simulink model "testmodel_5_clean"  (R2018b)
settings: Solver=VariableStepAuto  StartTime=0.0  StopTime=20  RelTol=1e-3
values from neighbouring files (symbols this model uses):
  Brain_gain = 3    [Model_versie_5_clean.m]
  Hoeksnelheid = 60    [Model_versie_1.m]    (also in Model_versie_5_clean.m = 200)
  k_1 = 1/K_g    (= 1.26582278481)    [Model_versie_1.m]    (also in Model_versie_5_clean.m)
  mu = 1.5    [Model_versie_1.m]    (also in Model_versie_5_clean.m = B_g/(2*sqrt(K_g*J_g)))
  Saccade_gain = 6    [Model_versie_5_clean.m]
  Time_delay = 0.00    (= 0)    [Model_versie_1.m]    (also in Model_versie_5_clean.m = 0.01)
  wn = 10    [Model_versie_1.m]    (also in Model_versie_5_clean.m = sqrt(K_g/J_g))
libraries: dspswit3 x1, simulink x1
settings Model: Creator=janwi  LastModifiedBy=janwi
settings SimscapeCC: SimscapeLogType=all

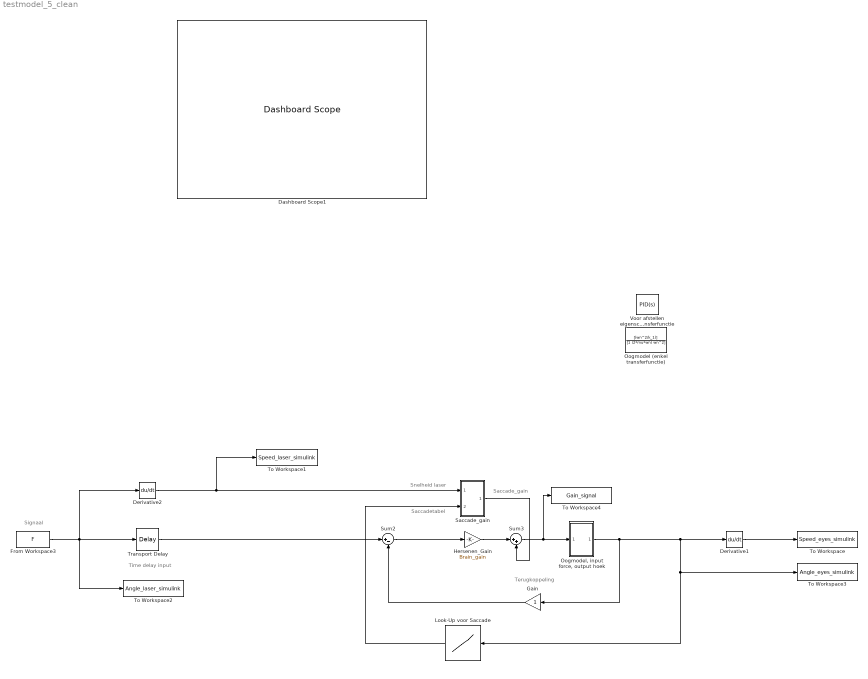
== system testmodel_5_clean ==
  note: Saccade_gain
  note: Saccadetabel
  note: Snelheid laser
  note: Terugkoppeling
  note: Signaal
  note: Time delay input
  Dashboard Scope1 : DashboardScope  WebBlockId=93
  Derivative1 : Derivative  CoefficientInTFapproximation=1
  Derivative2 : Derivative  CoefficientInTFapproximation=1
  From Workspace3 : FromWorkspace  VariableName=F  SampleTime=0
  Gain : Gain
  Hersenen_Gain : Gain  Gain=Brain_gain
  Look-Up voor Saccade : Lookup_n-D  NumberOfTableDimensions=1  BreakpointsForDimension1=[-34 -17 0 17 34]  Table=[1 2 3 2 1]  InternalRulePriority=Speed  RndMeth=Simplest  InputSameDT=on
  Oogmodel (enkel transferfunctie) : TransferFcn  Numerator=[(wn^2/k_1)]  Denominator=[1 (2*mu*wn) wn^2]
  "Oogmodel, input force, output hoek" : Subsystem
  Saccade_gain : Subsystem
  Sum2 : Sum  Inputs=|+-
  Sum3 : Sum  Inputs=|++
  To Workspace : ToWorkspace  VariableName=Speed_eyes_simulink  SampleTime=1e-3
      settings: Save2DSignal=2-D array (concatenate along first dimension)
  To Workspace1 : ToWorkspace  VariableName=Speed_laser_simulink  SampleTime=1e-3
      settings: Save2DSignal=2-D array (concatenate along first dimension)
  To Workspace2 : ToWorkspace  VariableName=Angle_laser_simulink  SampleTime=1e-3
      settings: Save2DSignal=2-D array (concatenate along first dimension)
  To Workspace3 : ToWorkspace  VariableName=Angle_eyes_simulink  SampleTime=1e-3
      settings: Save2DSignal=2-D array (concatenate along first dimension)
  To Workspace4 : ToWorkspace  VariableName=Gain_signal  SampleTime=1e-3
      settings: Save2DSignal=2-D array (concatenate along first dimension)
  Transport Delay : TransportDelay  DelayTime=Time_delay  InitialOutput=1
  Voor afstellen eigenschappen transferfunctie : simulink/Continuous/PID Controller  Controller=PID  Form=Parallel  TimeDomain=Continuous-time  SampleTime=-1  IntegratorMethod=Forward Euler  FilterMethod=Forward Euler  ControllerParametersSource=internal  P=2.20015768194357  I=166.043688229309  D=-0.000180470989757824  UseFilter=on  N=12191.1986236458  TunerSelectOption=Transfer Function Based (PID Tuner App)  InitialConditionSource=internal  InitialConditionForIntegrator=0  InitialConditionForFilter=0  DifferentiatorICPrevScaledInput=0  ExternalReset=none  TrackingMode=off  Kt=1  LimitOutput=off  UpperSaturationLimit=inf  LowerSaturationLimit=-inf  LinearizeAsGain=on  AntiWindupMode=none  Kb=1  POutMin=[]  POutMax=[]  IOutMin=[]  IOutMax=[]  DOutMin=[]  DOutMax=[]  NOutMin=[]  NOutMax=[]  SumOutMin=[]  SumOutMax=[]  SaturationOutMin=[]  SaturationOutMax=[]  PParamMin=[]  PParamMax=[]  IParamMin=[]  IParamMax=[]  DParamMin=[]  DParamMax=[]  NParamMin=[]  NParamMax=[]  KbParamMin=[]  KbParamMax=[]  KtParamMin=[]  KtParamMax=[]  KbOutMin=[]  KbOutMax=[]  KtOutMin=[]  KtOutMax=[]  IntegratorOutMin=[]  IntegratorOutMax=[]  FilterOutMin=[]  FilterOutMax=[]  SumI1OutMin=[]  SumI1OutMax=[]  SumI2OutMin=[]  SumI2OutMax=[]  SumI3OutMin=[]  SumI3OutMax=[]  SumI4OutMin=[]  SumI4OutMax=[]  SumDOutMin=[]  SumDOutMax=[]  DifferentiatorOutMin=[]  DifferentiatorOutMax=[]  FilterDiffOutCoefMin=[]  FilterDiffOutCoefMax=[]  ReciprocalOutMin=[]  ReciprocalOutMax=[]  SumDenOutMin=[]  SumDenOutMax=[]  SumNumOutMin=[]  SumNumOutMax=[]  DivideOutMin=[]  DivideOutMax=[]  IntegratorContinuousStateAttributes=''  IntegratorStateMustResolveToSignalObject=off  IntegratorRTWStateStorageClass=Auto  FilterContinuousStateAttributes=''  FilterStateMustResolveToSignalObject=off  FilterRTWStateStorageClass=Auto  ParallelPVariant=InternalParameters  IdealPVariant=Disabled  IVariant=InternalParameters  DVariant=InternalParameters  IntegratorVariant=Continuous  SatVariant=Disabled  AWVariant=Passthrough  PCopyVariant=Disabled  TRVariant=Disabled  FdbkBlocksVariant=Forward  IdealPFdbkVariant=Disabled  SatFdbkVariant=Disabled  DerivativeFilterVariant=ContFilter  NVariant=InternalParameters  NCopyVariant=Disabled  FilterICVariant=InternalICsFilter  IntegratorICVariant=InternalICs  ExternalResetVariant=Disabled  TRSumVariant=Passthrough  SumFdbkVariant=Disabled  SumVariant=Sum_PID
  wires:
  From Workspace3/1 -> To Workspace2/1, Transport Delay/1, Derivative2/1
  Derivative2/1 -> To Workspace1/1, Saccade_gain/1(In3)
  Transport Delay/1 -> Sum2/1
  Sum2/1 -> Hersenen_Gain/1
  "Oogmodel, input force, output hoek"/1(Out2) -> Look-Up voor Saccade/1, To Workspace3/1, Derivative1/1, Gain/1
  Derivative1/1 -> To Workspace/1
  Gain/1 -> Sum2/2
  Hersenen_Gain/1 -> Sum3/1
  Sum3/1 -> To Workspace4/1, "Oogmodel, input force, output hoek"/1(In1)
  Look-Up voor Saccade/1 -> Saccade_gain/2(In6)
  Saccade_gain/1(Out1) -> Sum3/2

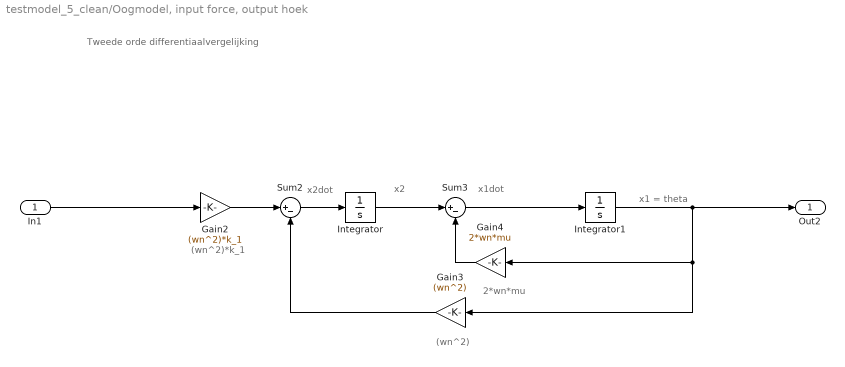
== system testmodel_5_clean/Oogmodel, input force, output hoek ==
  note: Tweede orde differentiaalvergelijking
  note: (wn^2)*k_1
  note: 2*wn*mu
  note: (wn^2)
  note: x2dot
  note: x2
  note: x1dot
  note: x1 = theta
  In1 : Inport
  Gain2 : Gain  Gain=(wn^2)*k_1
  Gain3 : Gain  Gain=(wn^2)
  Gain4 : Gain  Gain=2*wn*mu
  Integrator : Integrator
  Integrator1 : Integrator
  Sum2 : Sum  Inputs=|+-
  Sum3 : Sum  Inputs=|+-
  Out2 : Outport
  wires:
  Integrator1/1 -> Out2/1, Gain3/1, Gain4/1
  Gain3/1 -> Sum2/2
  Sum2/1 -> Integrator/1
  Gain2/1 -> Sum2/1
  Gain4/1 -> Sum3/2
  Integrator/1 -> Sum3/1
  Sum3/1 -> Integrator1/1
  In1/1 -> Gain2/1

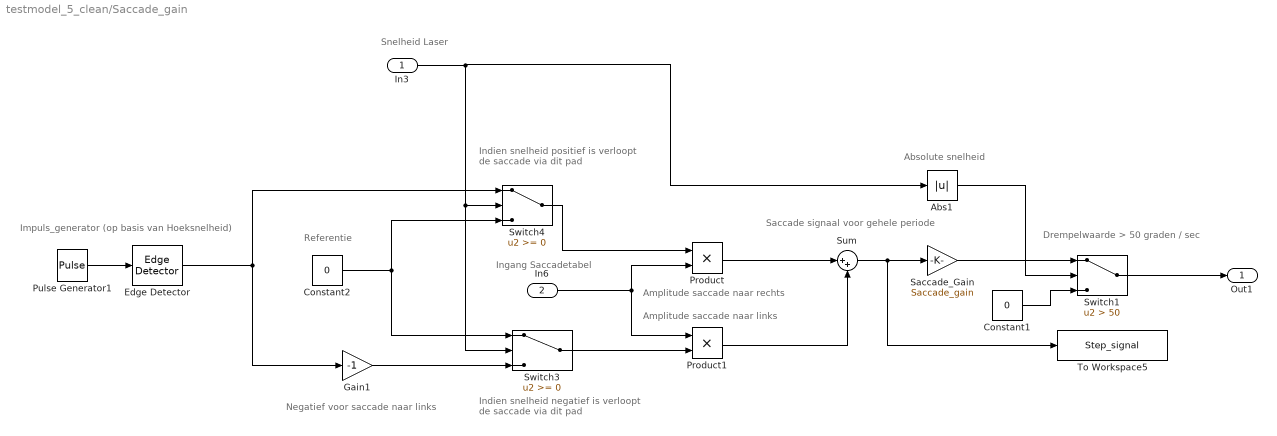
== system testmodel_5_clean/Saccade_gain ==
  note: Saccade signaal voor gehele periode
  note: Indien snelheid negatief
      | is verloopt de saccade via dit pad
  note: Negatief voor saccade naar links
  note: Referentie
  note: Impuls_generator (op basis van Hoeksnelheid)
  note: Amplitude saccade naar rechts
  note: Drempelwaarde > 50 graden / sec
  note: Absolute snelheid
  note: Snelheid Laser
  note: Ingang Saccadetabel
  note: Amplitude saccade naar links
  note: Indien snelheid positief
      | is verloopt de saccade via dit pad
  In3 : Inport
  In6 : Inport  Port=2
  Abs1 : Abs
  Constant1 : Constant  Value=0
  Constant2 : Constant  Value=0
  Edge Detector : dspswit3/Edge Detector  InputProcessing=Columns as channels (frame based)
      settings: SourceProductName=DSP System Toolbox  SourceProductBaseCode=DS
  Gain1 : Gain  Gain=-1
  Product : Product
  Product1 : Product
  Pulse Generator1 : DiscretePulseGenerator  PulseType=Time based  Period=1/(Hoeksnelheid/18)  PulseWidth=50
  Saccade_Gain : Gain  Gain=Saccade_gain
  Sum : Sum  Inputs=|++
  Switch1 : Switch  Criteria=u2 > Threshold  Threshold=50  ZeroCross=off
  Switch3 : Switch  ZeroCross=off
  Switch4 : Switch  ZeroCross=off
  To Workspace5 : ToWorkspace  VariableName=Step_signal  SampleTime=1e-3
      settings: Save2DSignal=2-D array (concatenate along first dimension)
  Out1 : Outport
  wires:
  Saccade_Gain/1 -> Switch1/1
  Abs1/1 -> Switch1/2
  Constant2/1 -> Switch4/3, Switch3/1
  In6/1 -> Product1/1, Product/2
  Switch3/1 -> Product1/2
  Constant1/1 -> Switch1/3
  Gain1/1 -> Switch3/3
  Sum/1 -> Saccade_Gain/1, To Workspace5/1
  Edge Detector/1 -> Gain1/1, Switch4/1
  In3/1 -> Abs1/1, Switch3/2, Switch4/2
  Pulse Generator1/1 -> Edge Detector/1
  Switch4/1 -> Product/1
  Product/1 -> Sum/1
  Product1/1 -> Sum/2
  Switch1/1 -> Out1/1
